simulink model "problem"  (R2016a)
settings: Solver=VariableStepAuto  StartTime=0.0  StopTime=10.0  RelTol=1e-3
libraries: simulink x1
settings Model: Creator=Mohammed Alaa Elkomy  LastModifiedBy=Mohammed Alaa Elkomy

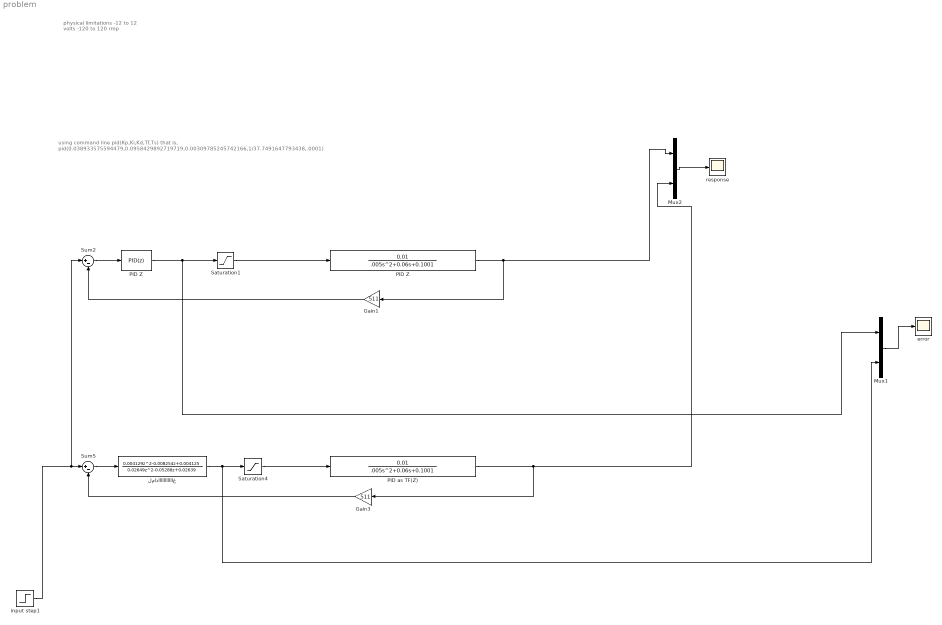
== system problem ==
  note: using command line
      | pid(Kp,Ki,Kd,Tf,Ts)
      | that is,
      | pid(0.038933575594479,0.0958429892719719,0.00309785245742166,1/37.7491647793438,.0001)
  note: physical limitations
      | -12 to 12 volts
      | -120 to 120 rmp
  Gain1 : Gain  Gain=511
  Gain3 : Gain  Gain=511
  Mux1 : Mux  Inputs=2
  Mux2 : Mux  Inputs=2
  PID Z : simulink/Continuous/PID Controller  Controller=PID  TimeDomain=Discrete-time  SampleTime=.0001  IntegratorMethod=Forward Euler  FilterMethod=Forward Euler  Form=Parallel  UseFilter=on  ControllerParametersSource=internal  P=0.038933575594479  I=0.0958429892719719  D=0.00309785245742166  N=37.7491647793438  InitialConditionSource=internal  InitialConditionForIntegrator=0  InitialConditionForFilter=0  ExternalReset=none  LimitOutput=off  UpperSaturationLimit=255  LowerSaturationLimit=0  LinearizeAsGain=on  AntiWindupMode=none  Kb=1  TrackingMode=off  Kt=1  PParamMin=[]  PParamMax=[]  IParamMin=[]  IParamMax=[]  DParamMin=[]  DParamMax=[]  NParamMin=[]  NParamMax=[]  KbParamMin=[]  KbParamMax=[]  KtParamMin=[]  KtParamMax=[]  POutMin=[]  POutMax=[]  IOutMin=[]  IOutMax=[]  DOutMin=[]  DOutMax=[]  NOutMin=[]  NOutMax=[]  KbOutMin=[]  KbOutMax=[]  KtOutMin=[]  KtOutMax=[]  IntegratorOutMin=[]  IntegratorOutMax=[]  FilterOutMin=[]  FilterOutMax=[]  SumOutMin=[]  SumOutMax=[]  SumI1OutMin=[]  SumI1OutMax=[]  SumI2OutMin=[]  SumI2OutMax=[]  SumI3OutMin=[]  SumI3OutMax=[]  SumDOutMin=[]  SumDOutMax=[]  SaturationOutMin=[]  SaturationOutMax=[]  IntegratorContinuousStateAttributes=''  IntegratorStateMustResolveToSignalObject=off  IntegratorRTWStateStorageClass=Auto  FilterContinuousStateAttributes=''  FilterStateMustResolveToSignalObject=off  FilterRTWStateStorageClass=Auto  DifferentiatorICPrevScaledInput=0  DifferentiatorOutMin=[]  DifferentiatorOutMax=[]
  "PID Z " : TransferFcn  Numerator=[0.01]  Denominator=[.005 0.06 0.1001]
  PID as TF(Z) : TransferFcn  Numerator=[0.01]  Denominator=[.005 0.06 0.1001]
  Saturation1 : Saturate  UpperLimit=255  LowerLimit=0
  Saturation4 : Saturate  UpperLimit=255  LowerLimit=0
  Sum2 : Sum  Inputs=|+-
  Sum5 : Sum  Inputs=|+-
  error : Scope
  input step1 : Step  Time=0  After=511  SampleTime=0
  response : Scope
  "لماذاااااااااااع " : DiscreteTransferFcn  Numerator="[0.004129  -0.008254   0.004125]"  Denominator="[ 0.02649   -0.05288   0.02639]"  SampleTime=.0001
  wires:
  Sum2/1 -> PID Z/1
  Gain1/1 -> Sum2/2
  Saturation1/1 -> "PID Z "/1
  "PID Z "/1 -> Mux2/1, Gain1/1
  Mux2/1 -> response/1
  Sum5/1 -> "لماذاااااااااااع "/1
  Gain3/1 -> Sum5/2
  Saturation4/1 -> PID as TF(Z)/1
  PID as TF(Z)/1 -> Mux2/2, Gain3/1
  input step1/1 -> Sum2/1, Sum5/1
  PID Z/1 -> Mux1/1, Saturation1/1
  Mux1/1 -> error/1
  "لماذاااااااااااع "/1 -> Mux1/2, Saturation4/1
